simulink model "MatlabClientTCPIPModel"  (R2016a)
settings: Solver=VariableStepAuto  StartTime=0.0  StopTime=10  RelTol=1e-3
settings Model: Creator=kalkadry  LastModifiedBy=kalkadry

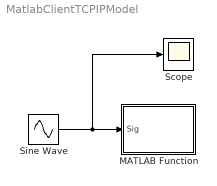
== system MatlabClientTCPIPModel ==
  MATLAB Function : MATLAB Function  TreatAsAtomicUnit=on
  Scope : Scope
  Sine Wave : Sin  SampleTime=0
  wires:
  Sine Wave/1 -> Scope/1, MATLAB Function/1(Sig)

== matlab function MatlabClientTCPIPModel/MATLAB Function ==
  data: Sig input
function fcn(Sig)
%#codegen

coder.extrinsic('tcpip');
coder.extrinsic('fwrite');
t = tcpip('localhost', 30000, 'NetworkRole', 'client');

fopen(t)

%Write the waveform to the server session.
fwrite(t, Sig)
